simulink model "sampleModel1887"  (R2023a)
settings: Solver=VariableStepAuto  StartTime=0.0  StopTime=10.0  RelTol=1e-3
libraries: hdlsllib x9, simulink x2
settings Model: Creator=user1  LastModifiedBy=user1

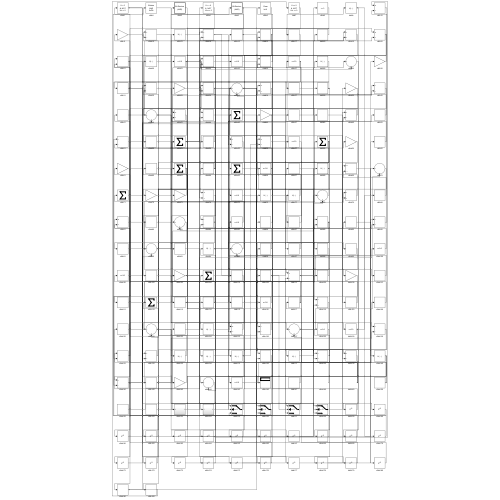
[thumbnail: Simulink's stored preview of the top-level diagram]
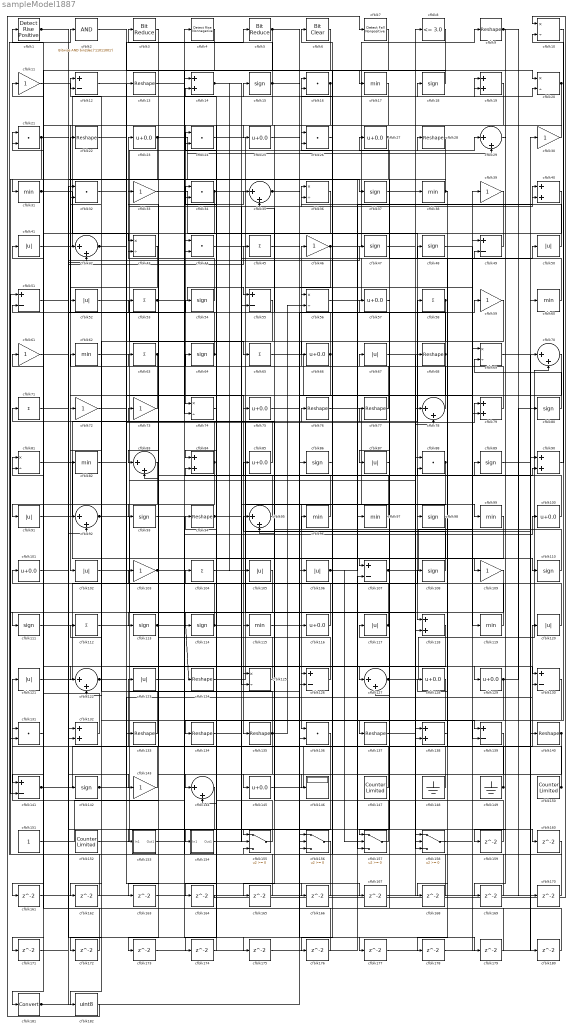
== system sampleModel1887 ==
  cfblk1 : hdlsllib/Logic and Bit Operations/Detect Rise Positive  vinit=0  OutDataTypeStr=boolean
  cfblk{10,20,36,43,56,69,74,81,125} (9 alike) : Product  Inputs=*/  RndMeth=Zero  SaturateOnIntegerOverflow=on
  cfblk{23,25,27,57,66,75,85,100..101,116,128..129,145} (13 alike) : Bias  Bias=0.0  SaturateOnIntegerOverflow=off
  cfblk{41,50,52,67,87,91,102,105..106,117,120..121,123} (13 alike) : Abs  SaturateOnIntegerOverflow=off
  cfblk{11,30,33,39,46,59,61,72..73,103,109,143} (12 alike) : Gain
  cfblk{45,53,58,63,65,71,104,112} (8 alike) : Sum  Inputs=+
  cfblk{12,49,51,55,107,126,130,139,141} (9 alike) : Sum  Inputs=+-
  cfblk{15,18,37,47..48,54,64,80,86,89,93,98,108,110..111,113..114,142} (18 alike) : Signum
  cfblk{17,31,38,60,62,82,96..97,99,115,119} (11 alike) : MinMax
  cfblk{14,19,40,79,84,90,118,132,138} (9 alike) : Sum
  cfblk{29,35,42,70,78,83,92,95,122,127,144} (11 alike) : Sum  Inputs=|++
  cfblk{9,13,22,28,68,76..77,94,124,133..135,137,140} (14 alike) : Reshape
  cfblk{16,21,24,26,32,34,44,88,131,136} (10 alike) : DotProduct  OutDataTypeStr=Inherit: Inherit via internal rule
  cfblk146 : Display
  cfblk147 : hdlsllib/Sources/Counter Limited  uplimit=7  tsamp=-1
  cfblk148 : Ground
  cfblk149 : Ground
  cfblk150 : hdlsllib/Sources/Counter Limited  uplimit=7  tsamp=-1
  cfblk151 : Constant  SampleTime=-1
  cfblk152 : hdlsllib/Sources/Counter Limited  uplimit=7  tsamp=-1
  cfblk153 : Subsystem
      settings: LibrarySourceBlock=|
      | hdlsllib/Ports &
      | Subsystems/Subsystem
  cfblk154 : Subsystem
      settings: LibrarySourceBlock=|
      | hdlsllib/Ports &
      | Subsystems/Subsystem
  cfblk{155..158} (4 alike) : Switch  SaturateOnIntegerOverflow=off  InputSameDT=off
  cfblk{159..180} (22 alike) : Delay  SampleTime=1
  cfblk181 : DataTypeConversion  SaturateOnIntegerOverflow=off  RndMeth=Floor
  cfblk182 : DataTypeConversion  OutDataTypeStr=uint8  SaturateOnIntegerOverflow=off  RndMeth=Floor
  cfblk2 : simulink/Logic and Bit Operations/Bitwise Operator  logicop=AND  UseBitMask=on  BitMask=bin2dec('11011001')  BitMaskRealWorld=Stored Integer
      settings: LibrarySourceBlock=|
      | hdlsllib/Logic and Bit
      | Operations/Bitwise
      | Operator
  cfblk3 : hdlsllib/Logic and Bit Operations/Bit Reduce  mode=AND
  cfblk4 : hdlsllib/Logic and Bit Operations/Detect Rise Nonnegative  vinit=0  OutDataTypeStr=boolean
  cfblk5 : hdlsllib/Logic and Bit Operations/Bit Reduce  mode=AND
  cfblk6 : simulink/Logic and Bit Operations/Bit Clear  iBit=0
      settings: LibrarySourceBlock=|
      | hdlsllib/Logic and Bit
      | Operations/Bit Clear
  cfblk7 : hdlsllib/Logic and Bit Operations/Detect Fall Nonpositive  vinit=0  OutDataTypeStr=boolean
  cfblk8 : hdlsllib/Logic and Bit Operations/Compare To Constant  relop=<=  const=3.0  OutDataTypeStr=boolean
  wires:
  cfblk142/1 -> cfblk36/1, cfblk130/2
  cfblk54/1 -> cfblk23/1
  cfblk133/1 -> cfblk101/1
  cfblk16/1 -> cfblk102/1, cfblk173/1
  cfblk98/1 -> cfblk136/1
  cfblk46/1 -> cfblk9/1, cfblk156/2
  cfblk18/1 -> cfblk17/1
  cfblk20/1 -> cfblk74/1, cfblk165/1
  cfblk41/1 -> cfblk18/1
  cfblk140/1 -> cfblk121/1, cfblk156/3, cfblk163/1
  cfblk15/1 -> cfblk3/1, cfblk20/2, cfblk144/2
  cfblk27/1 -> cfblk44/1, cfblk157/3
  cfblk76/1 -> cfblk99/1
  cfblk117/1 -> cfblk104/1, cfblk85/1
  cfblk10/1 -> cfblk137/1
  cfblk3/1 -> cfblk83/1
  cfblk82/1 -> cfblk155/1
  cfblk68/1 -> cfblk22/1, cfblk146/1
  cfblk87/1 -> cfblk67/1
  cfblk156/1 -> cfblk2/1
  cfblk79/1 -> cfblk46/1
  cfblk147/1 -> cfblk123/1
  cfblk70/1 -> cfblk135/1
  cfblk150/1 -> cfblk131/1, cfblk128/1
  cfblk63/1 -> cfblk122/2, cfblk172/1
  cfblk118/1 -> cfblk141/1
  cfblk158/1 -> cfblk69/1
  cfblk33/1 -> cfblk118/1
  cfblk85/1 -> cfblk34/1
  cfblk95/1 -> cfblk14/2
  cfblk143/1 -> cfblk81/1
  cfblk124/1 -> cfblk76/1
  cfblk155/1 -> cfblk94/1
  cfblk22/1 -> cfblk15/1
  cfblk21/1 -> cfblk37/1, cfblk141/2
  cfblk92/1 -> cfblk115/1, cfblk79/1
  cfblk88/1 -> cfblk126/1, cfblk125/2
  cfblk77/1 -> cfblk64/1
  cfblk62/1 -> cfblk16/1
  cfblk113/1 -> cfblk124/1, cfblk175/1
  cfblk35/1 -> cfblk130/1, cfblk79/2, cfblk167/1
  cfblk65/1 -> cfblk158/1
  cfblk50/1 -> cfblk26/1
  cfblk128/1 -> cfblk155/2
  cfblk8/1 -> cfblk66/1
  cfblk96/1 -> cfblk62/1
  cfblk31/1 -> cfblk43/1, cfblk179/1
  cfblk148/1 -> cfblk96/1
  cfblk24/1 -> cfblk98/1
  cfblk44/1 -> cfblk138/1
  cfblk127/1 -> cfblk70/2, cfblk89/1
  cfblk114/1 -> cfblk41/1, cfblk40/2
  cfblk149/1 -> cfblk117/1, cfblk57/1, cfblk53/1
  cfblk107/1 -> cfblk39/1, cfblk19/1
  cfblk138/1 -> cfblk48/1
  cfblk52/1 -> cfblk65/1
  cfblk119/1 -> cfblk12/1
  cfblk60/1 -> cfblk27/1
  cfblk14/1 -> cfblk109/1, cfblk105/1
  cfblk125/1 -> cfblk33/1
  cfblk73/1 -> cfblk72/1
  cfblk136/1 -> cfblk154/1(In1)
  cfblk122/1 -> cfblk158/2, cfblk166/1
  cfblk152/1 -> cfblk106/1
  cfblk80/1 -> cfblk69/2
  cfblk53/1 -> cfblk55/1, cfblk28/1, cfblk19/2
  cfblk105/1 -> cfblk134/1
  cfblk91/1 -> cfblk58/1
  cfblk13/1 -> cfblk4/1
  cfblk129/1 -> cfblk80/1, cfblk182/1
  cfblk11/1 -> cfblk12/2
  cfblk109/1 -> cfblk131/2
  cfblk26/1 -> cfblk6/1
  cfblk110/1 -> cfblk73/1
  cfblk132/1 -> cfblk51/2
  cfblk57/1 -> cfblk157/1
  cfblk28/1 -> cfblk87/1
  cfblk43/1 -> cfblk52/1
  cfblk47/1 -> cfblk29/1
  cfblk81/1 -> cfblk107/1
  cfblk9/1 -> cfblk169/1, cfblk170/1
  cfblk126/1 -> cfblk43/2
  cfblk45/1 -> cfblk139/1
  cfblk32/1 -> cfblk127/1
  cfblk108/1 -> cfblk95/1
  cfblk141/1 -> cfblk60/1, cfblk45/1
  cfblk103/1 -> cfblk138/2, cfblk35/1
  cfblk34/1 -> cfblk97/1, cfblk119/1, cfblk171/1
  cfblk111/1 -> cfblk88/1
  cfblk104/1 -> cfblk30/1
  cfblk97/1 -> cfblk56/1
  cfblk157/1 -> cfblk16/2
  cfblk112/1 -> cfblk108/1
  cfblk7/1 -> cfblk181/1
  cfblk4/1 -> cfblk83/2
  cfblk102/1 -> cfblk68/1
  cfblk116/1 -> cfblk103/1
  cfblk86/1 -> cfblk26/2
  cfblk144/1 -> cfblk153/1(In1)
  cfblk123/1 -> cfblk88/2
  cfblk121/1 -> cfblk13/1
  cfblk131/1 -> cfblk61/1
  cfblk51/1 -> cfblk142/1
  cfblk154/1(Out1) -> cfblk49/2
  cfblk39/1 -> cfblk55/2
  cfblk67/1 -> cfblk129/1
  cfblk37/1 -> cfblk38/1
  cfblk145/1 -> cfblk120/1
  cfblk120/1 -> cfblk71/1
  cfblk25/1 -> cfblk139/2
  cfblk30/1 -> cfblk25/1
  cfblk106/1 -> cfblk40/1, cfblk157/2
  cfblk115/1 -> cfblk59/1
  cfblk90/1 -> cfblk10/2
  cfblk55/1 -> cfblk113/1
  cfblk100/1 -> cfblk63/1
  cfblk84/1 -> cfblk111/1, cfblk11/1
  cfblk6/1 -> cfblk74/2
  cfblk101/1 -> cfblk54/1
  cfblk12/1 -> cfblk126/2
  cfblk40/1 -> cfblk132/2
  cfblk153/1(Out1) -> cfblk100/1
  cfblk36/1 -> cfblk84/1
  cfblk99/1 -> cfblk114/1
  cfblk42/1 -> cfblk133/1, cfblk75/1
  cfblk23/1 -> cfblk91/1, cfblk29/2, cfblk86/1
  cfblk69/1 -> cfblk140/1
  cfblk61/1 -> cfblk47/1
  cfblk137/1 -> cfblk78/1
  cfblk19/1 -> cfblk125/1
  cfblk49/1 -> cfblk42/1
  cfblk58/1 -> cfblk93/1, cfblk145/1, cfblk176/1
  cfblk135/1 -> cfblk112/1, cfblk144/1, cfblk56/2
  cfblk48/1 -> cfblk110/1
  cfblk151/1 -> cfblk44/2
  cfblk2/1 -> cfblk20/1
  cfblk38/1 -> cfblk31/1, cfblk178/1
  cfblk94/1 -> cfblk90/2, cfblk50/1
  cfblk59/1 -> cfblk82/1
  cfblk5/1 -> cfblk156/1, cfblk34/2
  cfblk64/1 -> cfblk24/1, cfblk21/1
  cfblk71/1 -> cfblk143/1
  cfblk134/1 -> cfblk77/1
  cfblk72/1 -> cfblk5/1
  cfblk56/1 -> cfblk8/1
  cfblk1/1 -> cfblk92/1, cfblk158/3
  cfblk66/1 -> cfblk122/1, cfblk35/2
  cfblk78/1 -> cfblk32/2
  cfblk29/1 -> cfblk159/1
  cfblk159/1 -> cfblk95/2
  cfblk93/1 -> cfblk160/1
  cfblk160/1 -> cfblk155/3
  cfblk17/1 -> cfblk161/1
  cfblk161/1 -> cfblk70/1
  cfblk83/1 -> cfblk162/1
  cfblk162/1 -> cfblk51/1
  cfblk163/1 -> cfblk78/2
  cfblk74/1 -> cfblk164/1
  cfblk164/1 -> cfblk10/1
  cfblk165/1 -> cfblk1/1
  cfblk166/1 -> cfblk81/2
  cfblk167/1 -> cfblk118/2
  cfblk130/1 -> cfblk168/1
  cfblk168/1 -> cfblk14/1
  cfblk169/1 -> cfblk32/1
  cfblk170/1 -> cfblk36/2
  cfblk171/1 -> cfblk42/2
  cfblk172/1 -> cfblk132/1
  cfblk173/1 -> cfblk107/2
  cfblk139/1 -> cfblk174/1
  cfblk174/1 -> cfblk84/2
  cfblk175/1 -> cfblk136/2
  cfblk176/1 -> cfblk24/2
  cfblk75/1 -> cfblk177/1
  cfblk177/1 -> cfblk49/1
  cfblk178/1 -> cfblk90/1
  cfblk179/1 -> cfblk21/2
  cfblk89/1 -> cfblk180/1
  cfblk180/1 -> cfblk127/2
  cfblk181/1 -> cfblk92/2, cfblk116/1
  cfblk182/1 -> cfblk7/1

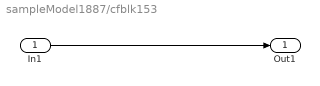
== system sampleModel1887/cfblk153 ==
  In1 : Inport
  Out1 : Outport
  wires:
  In1/1 -> Out1/1

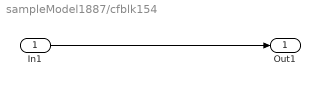
== system sampleModel1887/cfblk154 ==
  In1 : Inport
  Out1 : Outport
  wires:
  In1/1 -> Out1/1
